simulink model "SWC_HALOUT_type"  (R2021b)
settings: Solver=FixedStepDiscrete  StartTime=0.0  StopTime=10.0  FixedStep=0.005  RelTol=1e-3
undefined symbols (not defined in the file): DIDLen_APPD, DIDLen_APPE, DIDLen_APPPedalZP, DIDLen_APSFunConfig, DIDLen_AutoLock, DIDLen_AutoWipHSpdEN, DIDLen_CALID, DIDLen_CDEODT, DIDLen_CLRDIST, DIDLen_DKCBLESta, DIDLen_DKCKey, DIDLen_DKCSta, DIDLen_DoorNFCAnchorSta, DIDLen_DRLDis, DIDLen_DynoMode, DIDLen_ECUNAME, DIDLen_FDDKCCoordXY, DIDLen_FMHTimer, DIDLen_LFLowPresThre, DIDLen_LFSensorID, DIDLen_LIDAAnchorSta, DIDLen_LRLowPresThre, DIDLen_LRSensorID, DIDLen_MILDIST, DIDLen_NUMPSATRIPSFLTMEMCLR, DIDLen_NVMPedalZP, DIDLen_OBDReq, DIDLen_ODOMETER, DIDLen_PKE, DIDLen_ProtocolId, DIDLen_PSA, DIDLen_QTYPSATRIPS, DIDLen_RFLowPresThre, DIDLen_RFSensorID, DIDLen_RRLowPresThre, DIDLen_RRSensorID, DIDLen_RUNTM, DIDLen_SensorMode, DIDLen_TestGroup, DIDLen_TireSize, DIDLen_TPMSLearnSta, DIDLen_UIDSta, DIDLen_USSConfig, DIDLen_UWBAnchorSta, DIDLen_VIN, DIDLen_VSS, DIDLen_WhlPres, DIDLen_WhlSensorBattSta, DIDLen_WhlTmp, DIDLen_WipRLSCmdCutFilter, DIDLen_WipRLSCmdHoldFilter, DIDLen_XWDMode, DIDNum_APPD, DIDNum_APPE, DIDNum_APPPedalZP, DIDNum_APSFunConfig, DIDNum_AutoLock, DIDNum_AutoWipHSpdEN, DIDNum_CALID, DIDNum_CDEODT ... (+396)
libraries: simulink x213, FVT_lib x160, hdlsllib x6, hcu_lib x5, halout x1
(part 4 of 8)

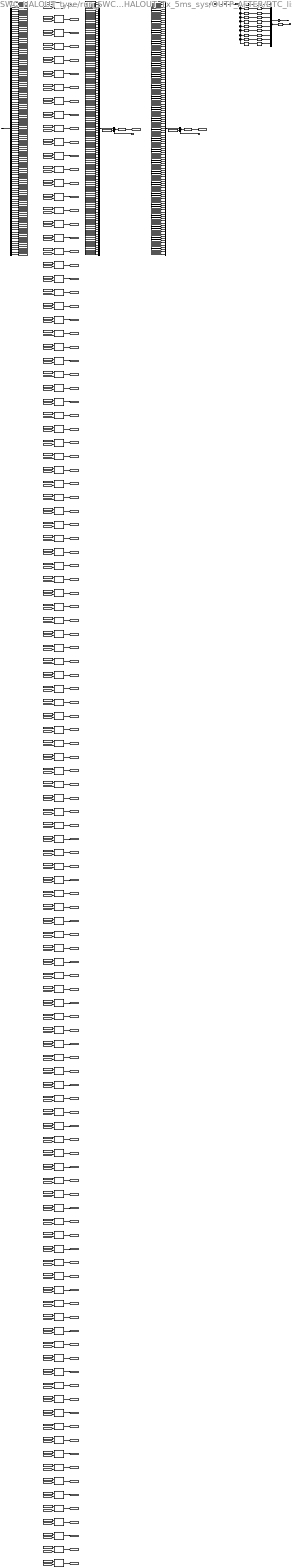
== system SWC_HALOUT_type/run_SWC_HALOUT_Tx_5ms_sys/OUTP_AFTER/DTC_list ==
  BOUTP_outputs : Inport
  BitwiseAND : simulink/Logic and Bit Operations/Bitwise Operator  logicop=AND  UseBitMask=on  BitMask=0x0001  BitMaskRealWorld=Stored Integer
  Constant : Constant  Value=DTC_D00201  OutDataTypeStr=uint16
  Constant1 : Constant  Value=DTC_D00202  OutDataTypeStr=uint16
  Constant10 : Constant  Value=DTC_10020B  OutDataTypeStr=uint16
  Constant100 : Constant  Value=DTC_900305  OutDataTypeStr=uint16
  Constant101 : Constant  Value=DTC_900253  OutDataTypeStr=uint16
  Constant102 : Constant  Value=DTC_900254  OutDataTypeStr=uint16
  Constant103 : Constant  Value=DTC_100A10  OutDataTypeStr=uint16
  Constant104 : Constant  Value=DTC_100A12  OutDataTypeStr=uint16
  Constant105 : Constant  Value=DTC_100A16  OutDataTypeStr=uint16
  Constant106 : Constant  Value=DTC_100A17  OutDataTypeStr=uint16
  Constant107 : Constant  Value=DTC_100A18  OutDataTypeStr=uint16
  Constant108 : Constant  Value=DTC_100A19  OutDataTypeStr=uint16
  Constant109 : Constant  Value=DTC_C0288F  OutDataTypeStr=uint16
  Constant11 : Constant  Value=DTC_10020C  OutDataTypeStr=uint16
  Constant110 : Constant  Value=DTC_C0378F  OutDataTypeStr=uint16
  Constant111 : Constant  Value=DTC_C0468F  OutDataTypeStr=uint16
  Constant112 : Constant  Value=DTC_C0558F  OutDataTypeStr=uint16
  Constant113 : Constant  Value=DTC_C0648F  OutDataTypeStr=uint16
  Constant114 : Constant  Value=DTC_C0808F  OutDataTypeStr=uint16
  Constant115 : Constant  Value=[0 0 0 0 0 0 0 0 0 0 0 0 0 0 0 0 0 0 0 0 0 0 0 0 0 0 0 0 0 0 0 0 0 0 0 0 0 0 0 0 0 0 0 0 0 0 0 0 0 0 0 0 0 0 0 0 0 0 0 0 0 0 0 0 0 0 0 0 0 0 0 0 0 0 0 0 0 0 0 0 0 0 0 0 0 0 0 0 0 0 0 0 0 0 0 0 0 0 0 0 0 0 0 0 0 0 0 0 0 0 0 0 0 0 0 0 0 0 0 0 0 0 0 0 0 0 0 0 0 0 0 0 0 0 0 0 0 0 0 0 0 0 0 0 0 0 0 0 0 0 0 0 0 0 0 0 0 0 0 0 0 0 0 0 0 0 0 0 0 0 0 0 0 0 0 0 0 0 0 0 0 0 0 0 0 0 0 0 0 0 0 0 0 0 0 0 0 0 0 0 0 0 0 0 0]  OutDataTypeStr=uint16
  Constant116 : DataTypeConversion
  Constant117 : Constant  Value=[0 0 0 0 0 0 0 0 0 0 0 0 0 0 0 0 0 0 0 0 0 0 0 0 0 0 0 0 0 0 0 0 0 0 0 0 0 0 0 0 0 0 0 0 0 0 0 0 0 0 0 0 0 0 0 0 0 0 0 0 0 0 0 0 0 0 0 0 0 0 0 0 0 0 0 0 0 0 0 0 0 0 0 0 0 0 0 0 0 0 0 0 0 0 0 0 0 0 0 0 0 0 0 0 0 0 0 0 0 0 0 0 0 0 0 0 0 0 0 0 0 0 0 0 0 0 0 0 0 0 0 0 0 0 0 0 0 0 0 0 0 0 0 0 0 0 0 0 0 0 0 0 0 0 0 0 0 0 0 0 0 0 0 0 0 0 0 0 0 0 0 0 0 0 0 0 0 0 0 0 0 0 0 0 0 0 0 0 0 0 0 0 0 0 0 0 0 0 0 0 0 0 0 0 0]  OutDataTypeStr=uint32
  Constant118 : DataTypeConversion
  Constant12 : Constant  Value=DTC_10020D  OutDataTypeStr=uint16
  Constant13 : Constant  Value=DTC_10020E  OutDataTypeStr=uint16
  Constant14 : Constant  Value=DTC_100210  OutDataTypeStr=uint16
  Constant15 : Constant  Value=DTC_100211  OutDataTypeStr=uint16
  Constant16 : Constant  Value=DTC_100212  OutDataTypeStr=uint16
  Constant17 : Constant  Value=DTC_100213  OutDataTypeStr=uint16
  Constant18 : Constant  Value=DTC_100214  OutDataTypeStr=uint16
  Constant19 : Constant  Value=DTC_100215  OutDataTypeStr=uint16
  Constant2 : Constant  Value=DTC_D00203  OutDataTypeStr=uint16
  Constant20 : Constant  Value=DTC_100216  OutDataTypeStr=uint16
  Constant21 : Constant  Value=DTC_100217  OutDataTypeStr=uint16
  Constant22 : Constant  Value=DTC_100218  OutDataTypeStr=uint16
  Constant23 : Constant  Value=DTC_100219  OutDataTypeStr=uint16
  Constant24 : Constant  Value=DTC_10021A  OutDataTypeStr=uint16
  Constant25 : Constant  Value=DTC_10021B  OutDataTypeStr=uint16
  Constant26 : Constant  Value=DTC_10021C  OutDataTypeStr=uint16
  Constant27 : Constant  Value=DTC_10021D  OutDataTypeStr=uint16
  Constant28 : Constant  Value=DTC_10021E  OutDataTypeStr=uint16
  Constant29 : Constant  Value=DTC_90021F  OutDataTypeStr=uint16
  Constant3 : Constant  Value=DTC_D00204  OutDataTypeStr=uint16
  Constant30 : Constant  Value=DTC_100220  OutDataTypeStr=uint16
  Constant31 : Constant  Value=DTC_100221  OutDataTypeStr=uint16
  Constant32 : Constant  Value=DTC_100223  OutDataTypeStr=uint16
  Constant33 : Constant  Value=DTC_100224  OutDataTypeStr=uint16
  Constant34 : Constant  Value=DTC_100225  OutDataTypeStr=uint16
  Constant35 : Constant  Value=DTC_100226  OutDataTypeStr=uint16
  Constant36 : Constant  Value=DTC_100227  OutDataTypeStr=uint16
  Constant37 : Constant  Value=DTC_D00228  OutDataTypeStr=uint16
  Constant38 : Constant  Value=DTC_D00229  OutDataTypeStr=uint16
  Constant39 : Constant  Value=DTC_D0022A  OutDataTypeStr=uint16
  Constant4 : Constant  Value=DTC_D00205  OutDataTypeStr=uint16
  Constant40 : Constant  Value=DTC_D0022B  OutDataTypeStr=uint16
  Constant41 : Constant  Value=DTC_D0022C  OutDataTypeStr=uint16
  Constant42 : Constant  Value=DTC_D0022D  OutDataTypeStr=uint16
  Constant43 : Constant  Value=DTC_90022F  OutDataTypeStr=uint16
  Constant44 : Constant  Value=DTC_D00230  OutDataTypeStr=uint16
  Constant45 : Constant  Value=DTC_D00231  OutDataTypeStr=uint16
  Constant46 : Constant  Value=DTC_D00232  OutDataTypeStr=uint16
  Constant47 : Constant  Value=DTC_D00234  OutDataTypeStr=uint16
  Constant48 : Constant  Value=DTC_D00235  OutDataTypeStr=uint16
  Constant49 : Constant  Value=DTC_D00236  OutDataTypeStr=uint16
  Constant5 : Constant  Value=DTC_D00206  OutDataTypeStr=uint16
  Constant50 : Constant  Value=DTC_D00237  OutDataTypeStr=uint16
  Constant51 : Constant  Value=DTC_D00238  OutDataTypeStr=uint16
  Constant52 : Constant  Value=DTC_D0023A  OutDataTypeStr=uint16
  Constant53 : Constant  Value=DTC_D0023B  OutDataTypeStr=uint16
  Constant54 : Constant  Value=DTC_D0023C  OutDataTypeStr=uint16
  Constant55 : Constant  Value=DTC_D0023D  OutDataTypeStr=uint16
  Constant56 : Constant  Value=DTC_D0023E  OutDataTypeStr=uint16
  Constant57 : Constant  Value=DTC_D00240  OutDataTypeStr=uint16
  Constant58 : Constant  Value=DTC_D00241  OutDataTypeStr=uint16
  Constant59 : Constant  Value=DTC_100242  OutDataTypeStr=uint16
  Constant6 : Constant  Value=DTC_D00207  OutDataTypeStr=uint16
  Constant60 : Constant  Value=DTC_100243  OutDataTypeStr=uint16
  Constant61 : Constant  Value=DTC_100244  OutDataTypeStr=uint16
  Constant62 : Constant  Value=DTC_100247  OutDataTypeStr=uint16
  Constant63 : Constant  Value=DTC_100248  OutDataTypeStr=uint16
  Constant64 : Constant  Value=DTC_100249  OutDataTypeStr=uint16
  Constant65 : Constant  Value=DTC_100250  OutDataTypeStr=uint16
  Constant66 : Constant  Value=DTC_100251  OutDataTypeStr=uint16
  Constant67 : Constant  Value=DTC_100252  OutDataTypeStr=uint16
  Constant68 : Constant  Value=DTC_900909  OutDataTypeStr=uint16
  Constant69 : Constant  Value=DTC_90090A  OutDataTypeStr=uint16
  Constant7 : Constant  Value=DTC_D00208  OutDataTypeStr=uint16
  Constant70 : Constant  Value=DTC_90090B  OutDataTypeStr=uint16
  Constant71 : Constant  Value=DTC_90090C  OutDataTypeStr=uint16
  Constant72 : Constant  Value=DTC_90090D  OutDataTypeStr=uint16
  Constant73 : Constant  Value=DTC_90090E  OutDataTypeStr=uint16
  Constant74 : Constant  Value=DTC_90090F  OutDataTypeStr=uint16
  Constant75 : Constant  Value=DTC_900910  OutDataTypeStr=uint16
  Constant76 : Constant  Value=DTC_900911  OutDataTypeStr=uint16
  Constant77 : Constant  Value=DTC_900912  OutDataTypeStr=uint16
  Constant78 : Constant  Value=DTC_900913  OutDataTypeStr=uint16
  Constant79 : Constant  Value=DTC_900914  OutDataTypeStr=uint16
  Constant8 : Constant  Value=DTC_D00209  OutDataTypeStr=uint16
  Constant80 : Constant  Value=DTC_500B01  OutDataTypeStr=uint16
  Constant81 : Constant  Value=DTC_500B02  OutDataTypeStr=uint16
  Constant82 : Constant  Value=DTC_500B03  OutDataTypeStr=uint16
  Constant83 : Constant  Value=DTC_500B04  OutDataTypeStr=uint16
  Constant84 : Constant  Value=DTC_500B05  OutDataTypeStr=uint16
  Constant85 : Constant  Value=DTC_500B06  OutDataTypeStr=uint16
  Constant86 : Constant  Value=DTC_500B07  OutDataTypeStr=uint16
  Constant87 : Constant  Value=DTC_500B08  OutDataTypeStr=uint16
  Constant88 : Constant  Value=DTC_500B09  OutDataTypeStr=uint16
  Constant89 : Constant  Value=DTC_500B0A  OutDataTypeStr=uint16
  Constant9 : Constant  Value=DTC_D0020A  OutDataTypeStr=uint16
  Constant90 : Constant  Value=DTC_500B0B  OutDataTypeStr=uint16
  Constant91 : Constant  Value=DTC_500B0C  OutDataTypeStr=uint16
  Constant92 : Constant  Value=DTC_500B0D  OutDataTypeStr=uint16
  Constant93 : Constant  Value=DTC_500B0E  OutDataTypeStr=uint16
  Constant94 : Constant  Value=DTC_500B0F  OutDataTypeStr=uint16
  Constant95 : Constant  Value=DTC_500B10  OutDataTypeStr=uint16
  Constant96 : Constant  Value=DTC_900301  OutDataTypeStr=uint16
  Constant97 : Constant  Value=DTC_900302  OutDataTypeStr=uint16
  Constant98 : Constant  Value=DTC_900303  OutDataTypeStr=uint16
  Constant99 : Constant  Value=DTC_900304  OutDataTypeStr=uint16
  DTCHeader{,1..9} (10 alike) : FVT_lib/hal/DTC_Header
  DTCID : Constant  Value=0xD00201
  DTCID+Status{,1..114} (115 alike) : FVT_lib/hal/DTC_ID_and_Info
  DTCID1 : Constant  Value=0xD00202
  DTCID10 : Constant  Value=0x10020B
  DTCID100 : Constant  Value=0x900305
  DTCID101 : Constant  Value=0x900253
  DTCID102 : Constant  Value=0x900254
  DTCID103 : Constant  Value=0x100A10
  DTCID104 : Constant  Value=0x100A12
  DTCID105 : Constant  Value=0x100A16
  DTCID106 : Constant  Value=0x100A17
  DTCID107 : Constant  Value=0x100A18
  DTCID108 : Constant  Value=0x100A19
  DTCID109 : Constant  Value=0xC0288F
  DTCID11 : Constant  Value=0x10020C
  DTCID110 : Constant  Value=0xC0378F
  DTCID111 : Constant  Value=0xC0468F
  DTCID112 : Constant  Value=0xC0558F
  DTCID113 : Constant  Value=0xC0648F
  DTCID114 : Constant  Value=0xC0808F
  DTCID12 : Constant  Value=0x10020D
  DTCID13 : Constant  Value=0x10020E
  DTCID14 : Constant  Value=0x100210
  DTCID15 : Constant  Value=0x100211
  DTCID16 : Constant  Value=0x100212
  DTCID17 : Constant  Value=0x100213
  DTCID18 : Constant  Value=0x100214
  DTCID19 : Constant  Value=0x100215
  DTCID2 : Constant  Value=0xD00203
  DTCID20 : Constant  Value=0x100216
  DTCID21 : Constant  Value=0x100217
  DTCID22 : Constant  Value=0x100218
  DTCID23 : Constant  Value=0x100219
  DTCID24 : Constant  Value=0x10021A
  DTCID25 : Constant  Value=0x10021B
  DTCID26 : Constant  Value=0x10021C
  DTCID27 : Constant  Value=0x10021D
  DTCID28 : Constant  Value=0x10021E
  DTCID29 : Constant  Value=0x90021F
  DTCID3 : Constant  Value=0xD00204
  DTCID30 : Constant  Value=0x100220
  DTCID31 : Constant  Value=0x100221
  DTCID32 : Constant  Value=0x100223
  DTCID33 : Constant  Value=0x100224
  DTCID34 : Constant  Value=0x100225
  DTCID35 : Constant  Value=0x100226
  DTCID36 : Constant  Value=0x100227
  DTCID37 : Constant  Value=0xD00228
  DTCID38 : Constant  Value=0xD00229
  DTCID39 : Constant  Value=0xD0022A
  DTCID4 : Constant  Value=0xD00205
  DTCID40 : Constant  Value=0xD0022B
  DTCID41 : Constant  Value=0xD0022C
  DTCID42 : Constant  Value=0xD0022D
  DTCID43 : Constant  Value=0x90022F
  DTCID44 : Constant  Value=0xD00230
  DTCID45 : Constant  Value=0xD00231
  DTCID46 : Constant  Value=0xD00232
  DTCID47 : Constant  Value=0xD00234
  DTCID48 : Constant  Value=0xD00235
  DTCID49 : Constant  Value=0xD00236
  DTCID5 : Constant  Value=0xD00206
  DTCID50 : Constant  Value=0xD00237
  DTCID51 : Constant  Value=0xD00238
  DTCID52 : Constant  Value=0xD0023A
  DTCID53 : Constant  Value=0xD0023B
  DTCID54 : Constant  Value=0xD0023C
  DTCID55 : Constant  Value=0xD0023D
  DTCID56 : Constant  Value=0xD0023E
  DTCID57 : Constant  Value=0xD00240
  DTCID58 : Constant  Value=0xD00241
  DTCID59 : Constant  Value=0x100242
  DTCID6 : Constant  Value=0xD00207
  DTCID60 : Constant  Value=0x100243
  DTCID61 : Constant  Value=0x100244
  DTCID62 : Constant  Value=0x100247
  DTCID63 : Constant  Value=0x100248
  DTCID64 : Constant  Value=0x100249
  DTCID65 : Constant  Value=0x100250
  DTCID66 : Constant  Value=0x100251
  DTCID67 : Constant  Value=0x100252
  DTCID68 : Constant  Value=0x900909
  DTCID69 : Constant  Value=0x90090A
  DTCID7 : Constant  Value=0xD00208
  DTCID70 : Constant  Value=0x90090B
  DTCID71 : Constant  Value=0x90090C
  DTCID72 : Constant  Value=0x90090D
  DTCID73 : Constant  Value=0x90090E
  DTCID74 : Constant  Value=0x90090F
  DTCID75 : Constant  Value=0x900910
  DTCID76 : Constant  Value=0x900911
  DTCID77 : Constant  Value=0x900912
  DTCID78 : Constant  Value=0x900913
  DTCID79 : Constant  Value=0x900914
  DTCID8 : Constant  Value=0xD00209
  DTCID80 : Constant  Value=0x500B01
  DTCID81 : Constant  Value=0x500B02
  DTCID82 : Constant  Value=0x500B03
  DTCID83 : Constant  Value=0x500B04
  DTCID84 : Constant  Value=0x500B05
  DTCID85 : Constant  Value=0x500B06
  DTCID86 : Constant  Value=0x500B07
  DTCID87 : Constant  Value=0x500B08
  DTCID88 : Constant  Value=0x500B09
  DTCID89 : Constant  Value=0x500B0A
  DTCID9 : Constant  Value=0xD0020A
  DTCID90 : Constant  Value=0x500B0B
  DTCID91 : Constant  Value=0x500B0C
  DTCID92 : Constant  Value=0x500B0D
  DTCID93 : Constant  Value=0x500B0E
  DTCID94 : Constant  Value=0x500B0F
  DTCID95 : Constant  Value=0x500B10
  DTCID96 : Constant  Value=0x900301
  DTCID97 : Constant  Value=0x900302
  DTCID98 : Constant  Value=0x900303
  DTCID99 : Constant  Value=0x900304
  Mux : Mux  Inputs=115
  Mux1 : Mux  Inputs=2
  Mux2 : Mux  Inputs=115
  Mux3 : Mux  Inputs=2
  Mux4 : Mux  Inputs=10
  OR : Logic  Operator=OR  Inputs=1  AllPortsSameDT=off  OutDataTypeStr=boolean
  Selector : Selector  InputPortWidth=320  IndexOptions=Index vector (dialog)  Indices=[1:32]  OutputSizes=1
  Selector1 : Selector  InputPortWidth=320  IndexOptions=Index vector (dialog)  Indices=[33:64]  OutputSizes=1
  Selector2 : Selector  InputPortWidth=320  IndexOptions=Index vector (dialog)  Indices=[65:96]  OutputSizes=1
  Selector3 : Selector  InputPortWidth=320  IndexOptions=Index vector (dialog)  Indices=[97:128]  OutputSizes=1
  Selector4 : Selector  InputPortWidth=320  IndexOptions=Index vector (dialog)  Indices=[129:160]  OutputSizes=1
  Selector5 : Selector  InputPortWidth=320  IndexOptions=Index vector (dialog)  Indices=[161:192]  OutputSizes=1
  Selector6 : Selector  InputPortWidth=320  IndexOptions=Index vector (dialog)  Indices=[193:224]  OutputSizes=1
  Selector7 : Selector  InputPortWidth=320  IndexOptions=Index vector (dialog)  Indices=[225:256]  OutputSizes=1
  Selector8 : Selector  InputPortWidth=320  IndexOptions=Index vector (dialog)  Indices=[257:288]  OutputSizes=1
  Selector9 : Selector  InputPortWidth=320  IndexOptions=Index vector (dialog)  Indices=[289:320]  OutputSizes=1
  UnitConverter : DataTypeConversion
  bus_selector : BusSelector  OutputSignals=VOUTP_5vAPS1PwrErrDTC_raw32,VOUTP_5vAPS2PwrErrDTC_raw32,VOUTP_ACCAccelCmdErrDetDTC_raw32,VOUTP_APS1SigOoRDTC_raw32,VOUTP_APS2SigOoRDTC_raw32,VOUTP_APSCorrErrDTC_raw32,VOUTP_BMSRdyDTC_raw32,VOUTP_BMSSigErrDetDTC_raw32,VOUTP_BrkSWErrDTC_raw32,VOUTP_BrkSWNoBacDTC_raw32,VOUTP_C1ABM1CSDTC_raw32,VOUTP_C1ABM1LCDTC_raw32,VOUTP_C1ABM1RCDTC_raw32,VOUTP_C3BMS1CSDTC_raw32,VOUTP_C3BMS1LCDTC_raw32,VOUTP_C3BMS1RCDTC_raw32,VOUTP_C3BMS6CSDTC_raw32,VOUTP_C3BMS6LCDTC_raw32,VOUTP_C3BMS6RCDTC_raw32,VOUTP_C3CCU1CSDTC_raw32,VOUTP_C3CCU1LCDTC_raw32,VOUTP_C3CCU1RCDTC_raw32,VOUTP_C3CCU2CSDTC_raw32,VOUTP_C3CCU2LCDTC_raw32,VOUTP_C3CCU2RCDTC_raw32,VOUTP_CAN1BusErrorDTC_raw32,VOUTP_CAN2BusErrorDTC_raw32,VOUTP_CAN3BusErrorDTC_raw32,VOUTP_CAN4BusErrorDTC_raw32,VOUTP_CAN5BusErrorDTC_raw32,VOUTP_CAN6BusErrorDTC_raw32,VOUTP_CCUSigErrDetDTC_raw32,VOUTP_DCDC4PreDTC_raw32,VOUTP_DCDCDisDTC_raw32,VOUTP_DCDCEnaDTC_raw32,VOUTP_DiagFLTSDTC_raw32,VOUTP_DiagFRTSDTC_raw32,VOUTP_DiagHCrashDTC_raw32,VOUTP_DiagRLTSDTC_raw32,VOUTP_DiagRRTSDTC_raw32,VOUTP_DrStSWDTC_raw32,VOUTP_EPBLockTODTC_raw32,VOUTP_EPBUnlockTODTC_raw32,VOUTP_ESC1CSErrDTC_raw32,VOUTP_ESC1NoComDTC_raw32,VOUTP_ESC1RCErrDTC_raw32,VOUTP_ESC5CSErrDTC_raw32,VOUTP_ESC5NoComDTC_raw32,VOUTP_ESC5RCErrDTC_raw32,VOUTP_FCLUSSDTC_raw32,VOUTP_FCMACCSigErrDetDTC_raw32,VOUTP_FCRUSSDTC_raw32,VOUTP_FLDoorSWDTC_raw32,VOUTP_FLLUSSDTC_raw32,VOUTP_FLRUSSDTC_raw32,VOUTP_FMLUSSDTC_raw32,VOUTP_FMRUSSDTC_raw32,VOUTP_FRDoorSWDTC_raw32,VOUTP_FrMCUSigErrDetDTC_raw32,VOUTP_FrMCUTqErrDTC_raw32,VOUTP_HVB4PreDTC_raw32,VOUTP_HVRlyCloDTC_raw32,VOUTP_HVRlyOpDTC_raw32,VOUTP_HiLvSaChkDTC_raw32,VOUTP_HoodSWDTC_raw32,VOUTP_IniLVLoDTC_raw32,VOUTP_KeyAuthDTC_raw32,VOUTP_LFBatwarnDTC_raw32,VOUTP_LFPressIndiDTC_raw32,VOUTP_LFSensorFailDTC_raw32,VOUTP_LFWheelTmpHighDTC_raw32,VOUTP_LRBatwarnDTC_raw32,VOUTP_LRPressIndiDTC_raw32,VOUTP_LRSensorFailDTC_raw32,VOUTP_LRWheelTmpHighDTC_raw32,VOUTP_LVSupHiDTC_raw32,VOUTP_LVSupLoDTC_raw32,VOUTP_Lv1ErrDTC_raw32,VOUTP_Lv2ErrDTC_raw32,VOUTP_Lv3ErrDTC_raw32,VOUTP_Lv4ErrDTC_raw32,VOUTP_MCU4PreDTC_raw32,VOUTP_MCUActDTC_raw32,VOUTP_MCUDisDTC_raw32,VOUTP_MCUF1CSErrDTC_raw32,VOUTP_MCUF1NoComDTC_raw32,VOUTP_MCUF1RCErrDTC_raw32,VOUTP_MCUR1CSErrDTC_raw32,VOUTP_MCUR1NoComDTC_raw32,VOUTP_MCUR1RCErrDTC_raw32,VOUTP_MidLvSaChkDTC_raw32,VOUTP_OBC4PreDTC_raw32,VOUTP_ONtoRdyDTC_raw32,VOUTP_RCLUSSDTC_raw32,VOUTP_RCRUSSDTC_raw32,VOUTP_RFBatwarnDTC_raw32,VOUTP_RFPressIndiDTC_raw32,VOUTP_RFSensorFailDTC_raw32,VOUTP_RFWheelTmpHighDTC_raw32,VOUTP_RLDoorSWDTC_raw32,VOUTP_RLLUSSDTC_raw32,VOUTP_RLRUSSDTC_raw32,VOUTP_RMLUSSDTC_raw32,VOUTP_RMRUSSDTC_raw32,VOUTP_RRBatwarnDTC_raw32,VOUTP_RRDoorSWDTC_raw32,VOUTP_RRPressIndiDTC_raw32,VOUTP_RRSensorFailDTC_raw32,VOUTP_RRWheelTmpHighDTC_raw32,VOUTP_RrMCUSigErrDetDTC_raw32,VOUTP_RrMCUTqErrDTC_raw32,VOUTP_Shifter1CSErrDTC_raw32,VOUTP_Shifter1NoComDTC_raw32,VOUTP_Shifter1RCErrDTC_raw32,VOUTP_TailgaSWDTC_raw32
  detect_change : simulink/Logic and Bit Operations/Detect Change  vinit=0  OutDataTypeStr=boolean
  Trigger : Outport
  Header_Array : Outport  Port=2
  DTC_Constant_Array : Outport  Port=3
  DTC_Array : Outport  Port=4
  wires:
  BOUTP_outputs/1 -> bus_selector/1
  bus_selector/1 -> [VOUTP_5vAPS1PwrErrDTC_raw32]  "<VOUTP_5vAPS1PwrErrDTC_raw32>"
  bus_selector/2 -> [VOUTP_5vAPS2PwrErrDTC_raw32]  "<VOUTP_5vAPS2PwrErrDTC_raw32>"
  bus_selector/3 -> [VOUTP_ACCAccelCmdErrDetDTC_raw32]  "<VOUTP_ACCAccelCmdErrDetDTC_raw32>"
  bus_selector/4 -> [VOUTP_APS1SigOoRDTC_raw32]  "<VOUTP_APS1SigOoRDTC_raw32>"
  bus_selector/5 -> [VOUTP_APS2SigOoRDTC_raw32]  "<VOUTP_APS2SigOoRDTC_raw32>"
  bus_selector/6 -> [VOUTP_APSCorrErrDTC_raw32]  "<VOUTP_APSCorrErrDTC_raw32>"
  bus_selector/7 -> [VOUTP_BMSRdyDTC_raw32]  "<VOUTP_BMSRdyDTC_raw32>"
  bus_selector/8 -> [VOUTP_BMSSigErrDetDTC_raw32]  "<VOUTP_BMSSigErrDetDTC_raw32>"
  bus_selector/9 -> [VOUTP_BrkSWErrDTC_raw32]  "<VOUTP_BrkSWErrDTC_raw32>"
  bus_selector/10 -> [VOUTP_BrkSWNoBacDTC_raw32]  "<VOUTP_BrkSWNoBacDTC_raw32>"
  bus_selector/11 -> [VOUTP_C1ABM1CSDTC_raw32]  "<VOUTP_C1ABM1CSDTC_raw32>"
  bus_selector/12 -> [VOUTP_C1ABM1LCDTC_raw32]  "<VOUTP_C1ABM1LCDTC_raw32>"
  bus_selector/13 -> [VOUTP_C1ABM1RCDTC_raw32]  "<VOUTP_C1ABM1RCDTC_raw32>"
  bus_selector/14 -> [VOUTP_C3BMS1CSDTC_raw32]  "<VOUTP_C3BMS1CSDTC_raw32>"
  bus_selector/15 -> [VOUTP_C3BMS1LCDTC_raw32]  "<VOUTP_C3BMS1LCDTC_raw32>"
  bus_selector/16 -> [VOUTP_C3BMS1RCDTC_raw32]  "<VOUTP_C3BMS1RCDTC_raw32>"
  bus_selector/17 -> [VOUTP_C3BMS6CSDTC_raw32]  "<VOUTP_C3BMS6CSDTC_raw32>"
  bus_selector/18 -> [VOUTP_C3BMS6LCDTC_raw32]  "<VOUTP_C3BMS6LCDTC_raw32>"
  bus_selector/19 -> [VOUTP_C3BMS6RCDTC_raw32]  "<VOUTP_C3BMS6RCDTC_raw32>"
  bus_selector/20 -> [VOUTP_C3CCU1CSDTC_raw32]  "<VOUTP_C3CCU1CSDTC_raw32>"
  bus_selector/21 -> [VOUTP_C3CCU1LCDTC_raw32]  "<VOUTP_C3CCU1LCDTC_raw32>"
  bus_selector/22 -> [VOUTP_C3CCU1RCDTC_raw32]  "<VOUTP_C3CCU1RCDTC_raw32>"
  bus_selector/23 -> [VOUTP_C3CCU2CSDTC_raw32]  "<VOUTP_C3CCU2CSDTC_raw32>"
  bus_selector/24 -> [VOUTP_C3CCU2LCDTC_raw32]  "<VOUTP_C3CCU2LCDTC_raw32>"
  bus_selector/25 -> [VOUTP_C3CCU2RCDTC_raw32]  "<VOUTP_C3CCU2RCDTC_raw32>"
  bus_selector/26 -> [VOUTP_CAN1BusErrorDTC_raw32]  "<VOUTP_CAN1BusErrorDTC_raw32>"
  bus_selector/27 -> [VOUTP_CAN2BusErrorDTC_raw32]  "<VOUTP_CAN2BusErrorDTC_raw32>"
  bus_selector/28 -> [VOUTP_CAN3BusErrorDTC_raw32]  "<VOUTP_CAN3BusErrorDTC_raw32>"
  bus_selector/29 -> [VOUTP_CAN4BusErrorDTC_raw32]  "<VOUTP_CAN4BusErrorDTC_raw32>"
  bus_selector/30 -> [VOUTP_CAN5BusErrorDTC_raw32]  "<VOUTP_CAN5BusErrorDTC_raw32>"
  bus_selector/31 -> [VOUTP_CAN6BusErrorDTC_raw32]  "<VOUTP_CAN6BusErrorDTC_raw32>"
  bus_selector/32 -> [VOUTP_CCUSigErrDetDTC_raw32]  "<VOUTP_CCUSigErrDetDTC_raw32>"
  bus_selector/33 -> [VOUTP_DCDC4PreDTC_raw32]  "<VOUTP_DCDC4PreDTC_raw32>"
  bus_selector/34 -> [VOUTP_DCDCDisDTC_raw32]  "<VOUTP_DCDCDisDTC_raw32>"
  bus_selector/35 -> [VOUTP_DCDCEnaDTC_raw32]  "<VOUTP_DCDCEnaDTC_raw32>"
  bus_selector/36 -> [VOUTP_DiagFLTSDTC_raw32]  "<VOUTP_DiagFLTSDTC_raw32>"
  bus_selector/37 -> [VOUTP_DiagFRTSDTC_raw32]  "<VOUTP_DiagFRTSDTC_raw32>"
  bus_selector/38 -> [VOUTP_DiagHCrashDTC_raw32]  "<VOUTP_DiagHCrashDTC_raw32>"
  bus_selector/39 -> [VOUTP_DiagRLTSDTC_raw32]  "<VOUTP_DiagRLTSDTC_raw32>"
  bus_selector/40 -> [VOUTP_DiagRRTSDTC_raw32]  "<VOUTP_DiagRRTSDTC_raw32>"
  bus_selector/41 -> [VOUTP_DrStSWDTC_raw32]  "<VOUTP_DrStSWDTC_raw32>"
  bus_selector/42 -> [VOUTP_EPBLockTODTC_raw32]  "<VOUTP_EPBLockTODTC_raw32>"
  bus_selector/43 -> [VOUTP_EPBUnlockTODTC_raw32]  "<VOUTP_EPBUnlockTODTC_raw32>"
  bus_selector/44 -> [VOUTP_ESC1CSErrDTC_raw32]  "<VOUTP_ESC1CSErrDTC_raw32>"
  bus_selector/45 -> [VOUTP_ESC1NoComDTC_raw32]  "<VOUTP_ESC1NoComDTC_raw32>"
  bus_selector/46 -> [VOUTP_ESC1RCErrDTC_raw32]  "<VOUTP_ESC1RCErrDTC_raw32>"
  bus_selector/47 -> [VOUTP_ESC5CSErrDTC_raw32]  "<VOUTP_ESC5CSErrDTC_raw32>"
  bus_selector/48 -> [VOUTP_ESC5NoComDTC_raw32]  "<VOUTP_ESC5NoComDTC_raw32>"
  bus_selector/49 -> [VOUTP_ESC5RCErrDTC_raw32]  "<VOUTP_ESC5RCErrDTC_raw32>"
  bus_selector/50 -> [VOUTP_FCLUSSDTC_raw32]  "<VOUTP_FCLUSSDTC_raw32>"
  bus_selector/51 -> [VOUTP_FCMACCSigErrDetDTC_raw32]  "<VOUTP_FCMACCSigErrDetDTC_raw32>"
  bus_selector/52 -> [VOUTP_FCRUSSDTC_raw32]  "<VOUTP_FCRUSSDTC_raw32>"
  bus_selector/53 -> [VOUTP_FLDoorSWDTC_raw32]  "<VOUTP_FLDoorSWDTC_raw32>"
  bus_selector/54 -> [VOUTP_FLLUSSDTC_raw32]  "<VOUTP_FLLUSSDTC_raw32>"
  bus_selector/55 -> [VOUTP_FLRUSSDTC_raw32]  "<VOUTP_FLRUSSDTC_raw32>"
  bus_selector/56 -> [VOUTP_FMLUSSDTC_raw32]  "<VOUTP_FMLUSSDTC_raw32>"
  bus_selector/57 -> [VOUTP_FMRUSSDTC_raw32]  "<VOUTP_FMRUSSDTC_raw32>"
  bus_selector/58 -> [VOUTP_FRDoorSWDTC_raw32]  "<VOUTP_FRDoorSWDTC_raw32>"
  bus_selector/59 -> [VOUTP_FrMCUSigErrDetDTC_raw32]  "<VOUTP_FrMCUSigErrDetDTC_raw32>"
  bus_selector/60 -> [VOUTP_FrMCUTqErrDTC_raw32]  "<VOUTP_FrMCUTqErrDTC_raw32>"
  bus_selector/61 -> [VOUTP_HVB4PreDTC_raw32]  "<VOUTP_HVB4PreDTC_raw32>"
  bus_selector/62 -> [VOUTP_HVRlyCloDTC_raw32]  "<VOUTP_HVRlyCloDTC_raw32>"
  bus_selector/63 -> [VOUTP_HVRlyOpDTC_raw32]  "<VOUTP_HVRlyOpDTC_raw32>"
  bus_selector/64 -> [VOUTP_HiLvSaChkDTC_raw32]  "<VOUTP_HiLvSaChkDTC_raw32>"
  bus_selector/65 -> [VOUTP_HoodSWDTC_raw32]  "<VOUTP_HoodSWDTC_raw32>"
  bus_selector/66 -> [VOUTP_IniLVLoDTC_raw32]  "<VOUTP_IniLVLoDTC_raw32>"
  bus_selector/67 -> [VOUTP_KeyAuthDTC_raw32]  "<VOUTP_KeyAuthDTC_raw32>"
  bus_selector/68 -> [VOUTP_LFBatwarnDTC_raw32]  "<VOUTP_LFBatwarnDTC_raw32>"
  bus_selector/69 -> [VOUTP_LFPressIndiDTC_raw32]  "<VOUTP_LFPressIndiDTC_raw32>"
  bus_selector/70 -> [VOUTP_LFSensorFailDTC_raw32]  "<VOUTP_LFSensorFailDTC_raw32>"
  bus_selector/71 -> [VOUTP_LFWheelTmpHighDTC_raw32]  "<VOUTP_LFWheelTmpHighDTC_raw32>"
  bus_selector/72 -> [VOUTP_LRBatwarnDTC_raw32]  "<VOUTP_LRBatwarnDTC_raw32>"
  bus_selector/73 -> [VOUTP_LRPressIndiDTC_raw32]  "<VOUTP_LRPressIndiDTC_raw32>"
  bus_selector/74 -> [VOUTP_LRSensorFailDTC_raw32]  "<VOUTP_LRSensorFailDTC_raw32>"
  bus_selector/75 -> [VOUTP_LRWheelTmpHighDTC_raw32]  "<VOUTP_LRWheelTmpHighDTC_raw32>"
  bus_selector/76 -> [VOUTP_LVSupHiDTC_raw32]  "<VOUTP_LVSupHiDTC_raw32>"
  bus_selector/77 -> [VOUTP_LVSupLoDTC_raw32]  "<VOUTP_LVSupLoDTC_raw32>"
  bus_selector/78 -> [VOUTP_Lv1ErrDTC_raw32]  "<VOUTP_Lv1ErrDTC_raw32>"
  bus_selector/79 -> [VOUTP_Lv2ErrDTC_raw32]  "<VOUTP_Lv2ErrDTC_raw32>"
  bus_selector/80 -> [VOUTP_Lv3ErrDTC_raw32]  "<VOUTP_Lv3ErrDTC_raw32>"
  bus_selector/81 -> [VOUTP_Lv4ErrDTC_raw32]  "<VOUTP_Lv4ErrDTC_raw32>"
  bus_selector/82 -> [VOUTP_MCU4PreDTC_raw32]  "<VOUTP_MCU4PreDTC_raw32>"
  bus_selector/83 -> [VOUTP_MCUActDTC_raw32]  "<VOUTP_MCUActDTC_raw32>"
  bus_selector/84 -> [VOUTP_MCUDisDTC_raw32]  "<VOUTP_MCUDisDTC_raw32>"
  bus_selector/85 -> [VOUTP_MCUF1CSErrDTC_raw32]  "<VOUTP_MCUF1CSErrDTC_raw32>"
  bus_selector/86 -> [VOUTP_MCUF1NoComDTC_raw32]  "<VOUTP_MCUF1NoComDTC_raw32>"
  bus_selector/87 -> [VOUTP_MCUF1RCErrDTC_raw32]  "<VOUTP_MCUF1RCErrDTC_raw32>"
  bus_selector/88 -> [VOUTP_MCUR1CSErrDTC_raw32]  "<VOUTP_MCUR1CSErrDTC_raw32>"
  bus_selector/89 -> [VOUTP_MCUR1NoComDTC_raw32]  "<VOUTP_MCUR1NoComDTC_raw32>"
  bus_selector/90 -> [VOUTP_MCUR1RCErrDTC_raw32]  "<VOUTP_MCUR1RCErrDTC_raw32>"
  bus_selector/91 -> [VOUTP_MidLvSaChkDTC_raw32]  "<VOUTP_MidLvSaChkDTC_raw32>"
  bus_selector/92 -> [VOUTP_OBC4PreDTC_raw32]  "<VOUTP_OBC4PreDTC_raw32>"
  bus_selector/93 -> [VOUTP_ONtoRdyDTC_raw32]  "<VOUTP_ONtoRdyDTC_raw32>"
  bus_selector/94 -> [VOUTP_RCLUSSDTC_raw32]  "<VOUTP_RCLUSSDTC_raw32>"
  bus_selector/95 -> [VOUTP_RCRUSSDTC_raw32]  "<VOUTP_RCRUSSDTC_raw32>"
  bus_selector/96 -> [VOUTP_RFBatwarnDTC_raw32]  "<VOUTP_RFBatwarnDTC_raw32>"
  bus_selector/97 -> [VOUTP_RFPressIndiDTC_raw32]  "<VOUTP_RFPressIndiDTC_raw32>"
  bus_selector/98 -> [VOUTP_RFSensorFailDTC_raw32]  "<VOUTP_RFSensorFailDTC_raw32>"
  bus_selector/99 -> [VOUTP_RFWheelTmpHighDTC_raw32]  "<VOUTP_RFWheelTmpHighDTC_raw32>"
  bus_selector/100 -> [VOUTP_RLDoorSWDTC_raw32]  "<VOUTP_RLDoorSWDTC_raw32>"
  bus_selector/101 -> [VOUTP_RLLUSSDTC_raw32]  "<VOUTP_RLLUSSDTC_raw32>"
  bus_selector/102 -> [VOUTP_RLRUSSDTC_raw32]  "<VOUTP_RLRUSSDTC_raw32>"
  bus_selector/103 -> [VOUTP_RMLUSSDTC_raw32]  "<VOUTP_RMLUSSDTC_raw32>"
  bus_selector/104 -> [VOUTP_RMRUSSDTC_raw32]  "<VOUTP_RMRUSSDTC_raw32>"
  bus_selector/105 -> [VOUTP_RRBatwarnDTC_raw32]  "<VOUTP_RRBatwarnDTC_raw32>"
  bus_selector/106 -> [VOUTP_RRDoorSWDTC_raw32]  "<VOUTP_RRDoorSWDTC_raw32>"
  bus_selector/107 -> [VOUTP_RRPressIndiDTC_raw32]  "<VOUTP_RRPressIndiDTC_raw32>"
  bus_selector/108 -> [VOUTP_RRSensorFailDTC_raw32]  "<VOUTP_RRSensorFailDTC_raw32>"
  bus_selector/109 -> [VOUTP_RRWheelTmpHighDTC_raw32]  "<VOUTP_RRWheelTmpHighDTC_raw32>"
  bus_selector/110 -> [VOUTP_RrMCUSigErrDetDTC_raw32]  "<VOUTP_RrMCUSigErrDetDTC_raw32>"
  bus_selector/111 -> [VOUTP_RrMCUTqErrDTC_raw32]  "<VOUTP_RrMCUTqErrDTC_raw32>"
  bus_selector/112 -> [VOUTP_Shifter1CSErrDTC_raw32]  "<VOUTP_Shifter1CSErrDTC_raw32>"
  bus_selector/113 -> [VOUTP_Shifter1NoComDTC_raw32]  "<VOUTP_Shifter1NoComDTC_raw32>"
  bus_selector/114 -> [VOUTP_Shifter1RCErrDTC_raw32]  "<VOUTP_Shifter1RCErrDTC_raw32>"
  bus_selector/115 -> [VOUTP_TailgaSWDTC_raw32]  "<VOUTP_TailgaSWDTC_raw32>"
  DTCID/1 -> DTCID+Status/1
  [VOUTP_C3BMS6RCDTC_raw32] -> DTCID+Status/2
  DTCID+Status/1 -> [DTC_raw0]
  DTCID1/1 -> DTCID+Status1/1
  [VOUTP_C3BMS6CSDTC_raw32] -> DTCID+Status1/2
  DTCID+Status1/1 -> [DTC_raw1]
  DTCID2/1 -> DTCID+Status2/1
  [VOUTP_C3BMS1RCDTC_raw32] -> DTCID+Status2/2
  DTCID+Status2/1 -> [DTC_raw2]
  DTCID3/1 -> DTCID+Status3/1
  [VOUTP_C3BMS1CSDTC_raw32] -> DTCID+Status3/2
  DTCID+Status3/1 -> [DTC_raw3]
  DTCID4/1 -> DTCID+Status4/1
  [VOUTP_C3CCU1RCDTC_raw32] -> DTCID+Status4/2
  DTCID+Status4/1 -> [DTC_raw4]
  DTCID5/1 -> DTCID+Status5/1
  [VOUTP_C3CCU1CSDTC_raw32] -> DTCID+Status5/2
  DTCID+Status5/1 -> [DTC_raw5]
  DTCID6/1 -> DTCID+Status6/1
  [VOUTP_C3CCU2RCDTC_raw32] -> DTCID+Status6/2
  DTCID+Status6/1 -> [DTC_raw6]
  DTCID7/1 -> DTCID+Status7/1
  [VOUTP_C3CCU2CSDTC_raw32] -> DTCID+Status7/2
  DTCID+Status7/1 -> [DTC_raw7]
  DTCID8/1 -> DTCID+Status8/1
  [VOUTP_C1ABM1RCDTC_raw32] -> DTCID+Status8/2
  DTCID+Status8/1 -> [DTC_raw8]
  DTCID9/1 -> DTCID+Status9/1
  [VOUTP_C1ABM1CSDTC_raw32] -> DTCID+Status9/2
  DTCID+Status9/1 -> [DTC_raw9]
  DTCID10/1 -> DTCID+Status10/1
  [VOUTP_Lv1ErrDTC_raw32] -> DTCID+Status10/2
  DTCID+Status10/1 -> [DTC_raw10]
  DTCID11/1 -> DTCID+Status11/1
  [VOUTP_Lv2ErrDTC_raw32] -> DTCID+Status11/2
  DTCID+Status11/1 -> [DTC_raw11]
  DTCID12/1 -> DTCID+Status12/1
  [VOUTP_Lv3ErrDTC_raw32] -> DTCID+Status12/2
  DTCID+Status12/1 -> [DTC_raw12]
  DTCID13/1 -> DTCID+Status13/1
  [VOUTP_Lv4ErrDTC_raw32] -> DTCID+Status13/2
  DTCID+Status13/1 -> [DTC_raw13]
  DTCID14/1 -> DTCID+Status14/1
  [VOUTP_IniLVLoDTC_raw32] -> DTCID+Status14/2
  DTCID+Status14/1 -> [DTC_raw14]
  DTCID15/1 -> DTCID+Status15/1
  [VOUTP_LVSupHiDTC_raw32] -> DTCID+Status15/2
  DTCID+Status15/1 -> [DTC_raw15]
  DTCID16/1 -> DTCID+Status16/1
  [VOUTP_LVSupLoDTC_raw32] -> DTCID+Status16/2
  DTCID+Status16/1 -> [DTC_raw16]
  DTCID17/1 -> DTCID+Status17/1
  [VOUTP_HVB4PreDTC_raw32] -> DTCID+Status17/2
  DTCID+Status17/1 -> [DTC_raw17]
  DTCID18/1 -> DTCID+Status18/1
  [VOUTP_MCU4PreDTC_raw32] -> DTCID+Status18/2
  DTCID+Status18/1 -> [DTC_raw18]
  DTCID19/1 -> DTCID+Status19/1
  [VOUTP_DCDC4PreDTC_raw32] -> DTCID+Status19/2
  DTCID+Status19/1 -> [DTC_raw19]
  DTCID20/1 -> DTCID+Status20/1
  [VOUTP_HVRlyCloDTC_raw32] -> DTCID+Status20/2
  DTCID+Status20/1 -> [DTC_raw20]
  DTCID21/1 -> DTCID+Status21/1
  [VOUTP_BMSRdyDTC_raw32] -> DTCID+Status21/2
  DTCID+Status21/1 -> [DTC_raw21]
  DTCID22/1 -> DTCID+Status22/1
  [VOUTP_DCDCEnaDTC_raw32] -> DTCID+Status22/2
  DTCID+Status22/1 -> [DTC_raw22]
  DTCID23/1 -> DTCID+Status23/1
  [VOUTP_HiLvSaChkDTC_raw32] -> DTCID+Status23/2
  DTCID+Status23/1 -> [DTC_raw23]
  DTCID24/1 -> DTCID+Status24/1
  [VOUTP_MidLvSaChkDTC_raw32] -> DTCID+Status24/2
  DTCID+Status24/1 -> [DTC_raw24]
  DTCID25/1 -> DTCID+Status25/1
  [VOUTP_MCUDisDTC_raw32] -> DTCID+Status25/2
  DTCID+Status25/1 -> [DTC_raw25]
  DTCID26/1 -> DTCID+Status26/1
  [VOUTP_DCDCDisDTC_raw32] -> DTCID+Status26/2
  DTCID+Status26/1 -> [DTC_raw26]
  DTCID27/1 -> DTCID+Status27/1
  [VOUTP_HVRlyOpDTC_raw32] -> DTCID+Status27/2
  DTCID+Status27/1 -> [DTC_raw27]
  DTCID28/1 -> DTCID+Status28/1
  [VOUTP_MCUActDTC_raw32] -> DTCID+Status28/2
  DTCID+Status28/1 -> [DTC_raw28]
  DTCID29/1 -> DTCID+Status29/1
  [VOUTP_OBC4PreDTC_raw32] -> DTCID+Status29/2
  DTCID+Status29/1 -> [DTC_raw29]
  DTCID30/1 -> DTCID+Status30/1
  [VOUTP_BrkSWErrDTC_raw32] -> DTCID+Status30/2
  DTCID+Status30/1 -> [DTC_raw30]
  DTCID31/1 -> DTCID+Status31/1
  [VOUTP_BrkSWNoBacDTC_raw32] -> DTCID+Status31/2
  DTCID+Status31/1 -> [DTC_raw31]
  DTCID32/1 -> DTCID+Status32/1
  [VOUTP_DrStSWDTC_raw32] -> DTCID+Status32/2
  DTCID+Status32/1 -> [DTC_raw32]
  DTCID33/1 -> DTCID+Status33/1
  [VOUTP_FLDoorSWDTC_raw32] -> DTCID+Status33/2
  DTCID+Status33/1 -> [DTC_raw33]
  DTCID34/1 -> DTCID+Status34/1
  [VOUTP_FRDoorSWDTC_raw32] -> DTCID+Status34/2
  DTCID+Status34/1 -> [DTC_raw34]
  DTCID35/1 -> DTCID+Status35/1
  [VOUTP_RLDoorSWDTC_raw32] -> DTCID+Status35/2
  DTCID+Status35/1 -> [DTC_raw35]
  DTCID36/1 -> DTCID+Status36/1
  [VOUTP_RRDoorSWDTC_raw32] -> DTCID+Status36/2
  DTCID+Status36/1 -> [DTC_raw36]
  DTCID37/1 -> DTCID+Status37/1
  [VOUTP_C3BMS6LCDTC_raw32] -> DTCID+Status37/2
  DTCID+Status37/1 -> [DTC_raw37]
  DTCID38/1 -> DTCID+Status38/1
  [VOUTP_C3BMS1LCDTC_raw32] -> DTCID+Status38/2
  DTCID+Status38/1 -> [DTC_raw38]
  DTCID39/1 -> DTCID+Status39/1
  [VOUTP_C3CCU1LCDTC_raw32] -> DTCID+Status39/2
  DTCID+Status39/1 -> [DTC_raw39]
  DTCID40/1 -> DTCID+Status40/1
  [VOUTP_C3CCU2LCDTC_raw32] -> DTCID+Status40/2
  DTCID+Status40/1 -> [DTC_raw40]
  DTCID41/1 -> DTCID+Status41/1
  [VOUTP_C1ABM1LCDTC_raw32] -> DTCID+Status41/2
  DTCID+Status41/1 -> [DTC_raw41]
  DTCID42/1 -> DTCID+Status42/1
  [VOUTP_KeyAuthDTC_raw32] -> DTCID+Status42/2
  DTCID+Status42/1 -> [DTC_raw42]
  DTCID43/1 -> DTCID+Status43/1
  [VOUTP_ONtoRdyDTC_raw32] -> DTCID+Status43/2
  DTCID+Status43/1 -> [DTC_raw43]
  DTCID44/1 -> DTCID+Status44/1
  [VOUTP_MCUR1NoComDTC_raw32] -> DTCID+Status44/2
  DTCID+Status44/1 -> [DTC_raw44]
  DTCID45/1 -> DTCID+Status45/1
  [VOUTP_MCUF1NoComDTC_raw32] -> DTCID+Status45/2
  DTCID+Status45/1 -> [DTC_raw45]
  DTCID46/1 -> DTCID+Status46/1
  [VOUTP_Shifter1NoComDTC_raw32] -> DTCID+Status46/2
  DTCID+Status46/1 -> [DTC_raw46]
  DTCID47/1 -> DTCID+Status47/1
  [VOUTP_ESC1NoComDTC_raw32] -> DTCID+Status47/2
  DTCID+Status47/1 -> [DTC_raw47]
  DTCID48/1 -> DTCID+Status48/1
  [VOUTP_ESC5NoComDTC_raw32] -> DTCID+Status48/2
  DTCID+Status48/1 -> [DTC_raw48]
  DTCID49/1 -> DTCID+Status49/1
  [VOUTP_MCUR1RCErrDTC_raw32] -> DTCID+Status49/2
  DTCID+Status49/1 -> [DTC_raw49]
  DTCID50/1 -> DTCID+Status50/1
  [VOUTP_MCUF1RCErrDTC_raw32] -> DTCID+Status50/2
  DTCID+Status50/1 -> [DTC_raw50]
  DTCID51/1 -> DTCID+Status51/1
  [VOUTP_Shifter1RCErrDTC_raw32] -> DTCID+Status51/2
  DTCID+Status51/1 -> [DTC_raw51]
  DTCID52/1 -> DTCID+Status52/1
  [VOUTP_ESC1RCErrDTC_raw32] -> DTCID+Status52/2
  DTCID+Status52/1 -> [DTC_raw52]
  DTCID53/1 -> DTCID+Status53/1
  [VOUTP_ESC5RCErrDTC_raw32] -> DTCID+Status53/2
  DTCID+Status53/1 -> [DTC_raw53]
  DTCID54/1 -> DTCID+Status54/1
  [VOUTP_MCUR1CSErrDTC_raw32] -> DTCID+Status54/2
  DTCID+Status54/1 -> [DTC_raw54]
  DTCID55/1 -> DTCID+Status55/1
  [VOUTP_MCUF1CSErrDTC_raw32] -> DTCID+Status55/2
  DTCID+Status55/1 -> [DTC_raw55]
  DTCID56/1 -> DTCID+Status56/1
  [VOUTP_Shifter1CSErrDTC_raw32] -> DTCID+Status56/2
  DTCID+Status56/1 -> [DTC_raw56]
  DTCID57/1 -> DTCID+Status57/1
  [VOUTP_ESC1CSErrDTC_raw32] -> DTCID+Status57/2
  DTCID+Status57/1 -> [DTC_raw57]
  DTCID58/1 -> DTCID+Status58/1
  [VOUTP_ESC5CSErrDTC_raw32] -> DTCID+Status58/2
  DTCID+Status58/1 -> [DTC_raw58]
  DTCID59/1 -> DTCID+Status59/1
  [VOUTP_APS1SigOoRDTC_raw32] -> DTCID+Status59/2
  DTCID+Status59/1 -> [DTC_raw59]
  DTCID60/1 -> DTCID+Status60/1
  [VOUTP_APS2SigOoRDTC_raw32] -> DTCID+Status60/2
  DTCID+Status60/1 -> [DTC_raw60]
  DTCID61/1 -> DTCID+Status61/1
  [VOUTP_APSCorrErrDTC_raw32] -> DTCID+Status61/2
  DTCID+Status61/1 -> [DTC_raw61]
  DTCID62/1 -> DTCID+Status62/1
  [VOUTP_5vAPS1PwrErrDTC_raw32] -> DTCID+Status62/2
  DTCID+Status62/1 -> [DTC_raw62]
  DTCID63/1 -> DTCID+Status63/1
  [VOUTP_5vAPS2PwrErrDTC_raw32] -> DTCID+Status63/2
  DTCID+Status63/1 -> [DTC_raw63]
  DTCID64/1 -> DTCID+Status64/1
  [VOUTP_FrMCUTqErrDTC_raw32] -> DTCID+Status64/2
  DTCID+Status64/1 -> [DTC_raw64]
  DTCID65/1 -> DTCID+Status65/1
  [VOUTP_RrMCUTqErrDTC_raw32] -> DTCID+Status65/2
  DTCID+Status65/1 -> [DTC_raw65]
  DTCID66/1 -> DTCID+Status66/1
  [VOUTP_EPBLockTODTC_raw32] -> DTCID+Status66/2
  DTCID+Status66/1 -> [DTC_raw66]
  DTCID67/1 -> DTCID+Status67/1
  [VOUTP_EPBUnlockTODTC_raw32] -> DTCID+Status67/2
  DTCID+Status67/1 -> [DTC_raw67]
  DTCID68/1 -> DTCID+Status68/1
  [VOUTP_FCLUSSDTC_raw32] -> DTCID+Status68/2
  DTCID+Status68/1 -> [DTC_raw68]
  DTCID69/1 -> DTCID+Status69/1
  [VOUTP_FMLUSSDTC_raw32] -> DTCID+Status69/2
  DTCID+Status69/1 -> [DTC_raw69]
  DTCID70/1 -> DTCID+Status70/1
  [VOUTP_FMRUSSDTC_raw32] -> DTCID+Status70/2
  DTCID+Status70/1 -> [DTC_raw70]
  DTCID71/1 -> DTCID+Status71/1
  [VOUTP_FCRUSSDTC_raw32] -> DTCID+Status71/2
  DTCID+Status71/1 -> [DTC_raw71]
  DTCID72/1 -> DTCID+Status72/1
  [VOUTP_RCLUSSDTC_raw32] -> DTCID+Status72/2
  DTCID+Status72/1 -> [DTC_raw72]
  DTCID73/1 -> DTCID+Status73/1
  [VOUTP_RMLUSSDTC_raw32] -> DTCID+Status73/2
  DTCID+Status73/1 -> [DTC_raw73]
  DTCID74/1 -> DTCID+Status74/1
  [VOUTP_RMRUSSDTC_raw32] -> DTCID+Status74/2
  DTCID+Status74/1 -> [DTC_raw74]
  DTCID75/1 -> DTCID+Status75/1
  [VOUTP_RCRUSSDTC_raw32] -> DTCID+Status75/2
  DTCID+Status75/1 -> [DTC_raw75]
  DTCID76/1 -> DTCID+Status76/1
  [VOUTP_FLLUSSDTC_raw32] -> DTCID+Status76/2
  DTCID+Status76/1 -> [DTC_raw76]
  DTCID77/1 -> DTCID+Status77/1
  [VOUTP_FLRUSSDTC_raw32] -> DTCID+Status77/2
  DTCID+Status77/1 -> [DTC_raw77]
  DTCID78/1 -> DTCID+Status78/1
  [VOUTP_RLLUSSDTC_raw32] -> DTCID+Status78/2
  DTCID+Status78/1 -> [DTC_raw78]
  DTCID79/1 -> DTCID+Status79/1
  [VOUTP_RLRUSSDTC_raw32] -> DTCID+Status79/2
  DTCID+Status79/1 -> [DTC_raw79]
  DTCID80/1 -> DTCID+Status80/1
  [VOUTP_LFPressIndiDTC_raw32] -> DTCID+Status80/2
  DTCID+Status80/1 -> [DTC_raw80]
  DTCID81/1 -> DTCID+Status81/1
  [VOUTP_RFPressIndiDTC_raw32] -> DTCID+Status81/2
  DTCID+Status81/1 -> [DTC_raw81]
  DTCID82/1 -> DTCID+Status82/1
  [VOUTP_LRPressIndiDTC_raw32] -> DTCID+Status82/2
  DTCID+Status82/1 -> [DTC_raw82]
  DTCID83/1 -> DTCID+Status83/1
  [VOUTP_RRPressIndiDTC_raw32] -> DTCID+Status83/2
  DTCID+Status83/1 -> [DTC_raw83]
  DTCID84/1 -> DTCID+Status84/1
  [VOUTP_LFWheelTmpHighDTC_raw32] -> DTCID+Status84/2
  DTCID+Status84/1 -> [DTC_raw84]
  DTCID85/1 -> DTCID+Status85/1
  [VOUTP_RFWheelTmpHighDTC_raw32] -> DTCID+Status85/2
  DTCID+Status85/1 -> [DTC_raw85]
  DTCID86/1 -> DTCID+Status86/1
  [VOUTP_LRWheelTmpHighDTC_raw32] -> DTCID+Status86/2
  DTCID+Status86/1 -> [DTC_raw86]
  DTCID87/1 -> DTCID+Status87/1
  [VOUTP_RRWheelTmpHighDTC_raw32] -> DTCID+Status87/2
  DTCID+Status87/1 -> [DTC_raw87]
  DTCID88/1 -> DTCID+Status88/1
  [VOUTP_LFBatwarnDTC_raw32] -> DTCID+Status88/2
  DTCID+Status88/1 -> [DTC_raw88]
  DTCID89/1 -> DTCID+Status89/1
  [VOUTP_RFBatwarnDTC_raw32] -> DTCID+Status89/2
  DTCID+Status89/1 -> [DTC_raw89]
  DTCID90/1 -> DTCID+Status90/1
  [VOUTP_LRBatwarnDTC_raw32] -> DTCID+Status90/2
  DTCID+Status90/1 -> [DTC_raw90]
  DTCID91/1 -> DTCID+Status91/1
  [VOUTP_RRBatwarnDTC_raw32] -> DTCID+Status91/2
  DTCID+Status91/1 -> [DTC_raw91]
  DTCID92/1 -> DTCID+Status92/1
  [VOUTP_LFSensorFailDTC_raw32] -> DTCID+Status92/2
  DTCID+Status92/1 -> [DTC_raw92]
  DTCID93/1 -> DTCID+Status93/1
  [VOUTP_RFSensorFailDTC_raw32] -> DTCID+Status93/2
  DTCID+Status93/1 -> [DTC_raw93]
  DTCID94/1 -> DTCID+Status94/1
  [VOUTP_LRSensorFailDTC_raw32] -> DTCID+Status94/2
  DTCID+Status94/1 -> [DTC_raw94]
  DTCID95/1 -> DTCID+Status95/1
  [VOUTP_RRSensorFailDTC_raw32] -> DTCID+Status95/2
  DTCID+Status95/1 -> [DTC_raw95]
  DTCID96/1 -> DTCID+Status96/1
  [VOUTP_DiagFRTSDTC_raw32] -> DTCID+Status96/2
  DTCID+Status96/1 -> [DTC_raw96]
  DTCID97/1 -> DTCID+Status97/1
  [VOUTP_DiagRRTSDTC_raw32] -> DTCID+Status97/2
  DTCID+Status97/1 -> [DTC_raw97]
  DTCID98/1 -> DTCID+Status98/1
  [VOUTP_DiagFLTSDTC_raw32] -> DTCID+Status98/2
  DTCID+Status98/1 -> [DTC_raw98]
  DTCID99/1 -> DTCID+Status99/1
  [VOUTP_DiagRLTSDTC_raw32] -> DTCID+Status99/2
  DTCID+Status99/1 -> [DTC_raw99]
  DTCID100/1 -> DTCID+Status100/1
  [VOUTP_DiagHCrashDTC_raw32] -> DTCID+Status100/2
  DTCID+Status100/1 -> [DTC_raw100]
  DTCID101/1 -> DTCID+Status101/1
  [VOUTP_HoodSWDTC_raw32] -> DTCID+Status101/2
  DTCID+Status101/1 -> [DTC_raw101]
  DTCID102/1 -> DTCID+Status102/1
  [VOUTP_TailgaSWDTC_raw32] -> DTCID+Status102/2
  DTCID+Status102/1 -> [DTC_raw102]
  DTCID103/1 -> DTCID+Status103/1
  [VOUTP_BMSSigErrDetDTC_raw32] -> DTCID+Status103/2
  DTCID+Status103/1 -> [DTC_raw103]
  DTCID104/1 -> DTCID+Status104/1
  [VOUTP_FCMACCSigErrDetDTC_raw32] -> DTCID+Status104/2
  DTCID+Status104/1 -> [DTC_raw104]
  DTCID105/1 -> DTCID+Status105/1
  [VOUTP_FrMCUSigErrDetDTC_raw32] -> DTCID+Status105/2
  DTCID+Status105/1 -> [DTC_raw105]
  DTCID106/1 -> DTCID+Status106/1
  [VOUTP_RrMCUSigErrDetDTC_raw32] -> DTCID+Status106/2
  DTCID+Status106/1 -> [DTC_raw106]
  DTCID107/1 -> DTCID+Status107/1
  [VOUTP_CCUSigErrDetDTC_raw32] -> DTCID+Status107/2
  DTCID+Status107/1 -> [DTC_raw107]
  DTCID108/1 -> DTCID+Status108/1
  [VOUTP_ACCAccelCmdErrDetDTC_raw32] -> DTCID+Status108/2
  DTCID+Status108/1 -> [DTC_raw108]
  DTCID109/1 -> DTCID+Status109/1
  [VOUTP_CAN1BusErrorDTC_raw32] -> DTCID+Status109/2
  DTCID+Status109/1 -> [DTC_raw109]
  DTCID110/1 -> DTCID+Status110/1
  [VOUTP_CAN2BusErrorDTC_raw32] -> DTCID+Status110/2
  DTCID+Status110/1 -> [DTC_raw110]
  DTCID111/1 -> DTCID+Status111/1
  [VOUTP_CAN3BusErrorDTC_raw32] -> DTCID+Status111/2
  DTCID+Status111/1 -> [DTC_raw111]
  DTCID112/1 -> DTCID+Status112/1
  [VOUTP_CAN4BusErrorDTC_raw32] -> DTCID+Status112/2
  DTCID+Status112/1 -> [DTC_raw112]
  DTCID113/1 -> DTCID+Status113/1
  [VOUTP_CAN5BusErrorDTC_raw32] -> DTCID+Status113/2
  DTCID+Status113/1 -> [DTC_raw113]
  DTCID114/1 -> DTCID+Status114/1
  [VOUTP_CAN6BusErrorDTC_raw32] -> DTCID+Status114/2
  DTCID+Status114/1 -> [DTC_raw114]
  Constant/1 -> Mux/1
  Constant1/1 -> Mux/2
  Constant2/1 -> Mux/3
  Constant3/1 -> Mux/4
  Constant4/1 -> Mux/5
  Constant5/1 -> Mux/6
  Constant6/1 -> Mux/7
  Constant7/1 -> Mux/8
  Constant8/1 -> Mux/9
  Constant9/1 -> Mux/10
  Constant10/1 -> Mux/11
  Constant11/1 -> Mux/12
  Constant12/1 -> Mux/13
  Constant13/1 -> Mux/14
  Constant14/1 -> Mux/15
  Constant15/1 -> Mux/16
  Constant16/1 -> Mux/17
  Constant17/1 -> Mux/18
  Constant18/1 -> Mux/19
  Constant19/1 -> Mux/20
  Constant20/1 -> Mux/21
  Constant21/1 -> Mux/22
  Constant22/1 -> Mux/23
  Constant23/1 -> Mux/24
  Constant24/1 -> Mux/25
  Constant25/1 -> Mux/26
  Constant26/1 -> Mux/27
  Constant27/1 -> Mux/28
  Constant28/1 -> Mux/29
  Constant29/1 -> Mux/30
  Constant30/1 -> Mux/31
  Constant31/1 -> Mux/32
  Constant32/1 -> Mux/33
  Constant33/1 -> Mux/34
  Constant34/1 -> Mux/35
  Constant35/1 -> Mux/36
  Constant36/1 -> Mux/37
  Constant37/1 -> Mux/38
  Constant38/1 -> Mux/39
  Constant39/1 -> Mux/40
  Constant40/1 -> Mux/41
  Constant41/1 -> Mux/42
  Constant42/1 -> Mux/43
  Constant43/1 -> Mux/44
  Constant44/1 -> Mux/45
  Constant45/1 -> Mux/46
  Constant46/1 -> Mux/47
  Constant47/1 -> Mux/48
  Constant48/1 -> Mux/49
  Constant49/1 -> Mux/50
  Constant50/1 -> Mux/51
  Constant51/1 -> Mux/52
  Constant52/1 -> Mux/53
  Constant53/1 -> Mux/54
  Constant54/1 -> Mux/55
  Constant55/1 -> Mux/56
  Constant56/1 -> Mux/57
  Constant57/1 -> Mux/58
  Constant58/1 -> Mux/59
  Constant59/1 -> Mux/60
  Constant60/1 -> Mux/61
  Constant61/1 -> Mux/62
  Constant62/1 -> Mux/63
  Constant63/1 -> Mux/64
  Constant64/1 -> Mux/65
  Constant65/1 -> Mux/66
  Constant66/1 -> Mux/67
  Constant67/1 -> Mux/68
  Constant68/1 -> Mux/69
  Constant69/1 -> Mux/70
  Constant70/1 -> Mux/71
  Constant71/1 -> Mux/72
  Constant72/1 -> Mux/73
  Constant73/1 -> Mux/74
  Constant74/1 -> Mux/75
  Constant75/1 -> Mux/76
  Constant76/1 -> Mux/77
  Constant77/1 -> Mux/78
  Constant78/1 -> Mux/79
  Constant79/1 -> Mux/80
  Constant80/1 -> Mux/81
  Constant81/1 -> Mux/82
  Constant82/1 -> Mux/83
  Constant83/1 -> Mux/84
  Constant84/1 -> Mux/85
  Constant85/1 -> Mux/86
  Constant86/1 -> Mux/87
  Constant87/1 -> Mux/88
  Constant88/1 -> Mux/89
  Constant89/1 -> Mux/90
  Constant90/1 -> Mux/91
  Constant91/1 -> Mux/92
  Constant92/1 -> Mux/93
  Constant93/1 -> Mux/94
  Constant94/1 -> Mux/95
  Constant95/1 -> Mux/96
  Constant96/1 -> Mux/97
  Constant97/1 -> Mux/98
  Constant98/1 -> Mux/99
  Constant99/1 -> Mux/100
  Constant100/1 -> Mux/101
  Constant101/1 -> Mux/102
  Constant102/1 -> Mux/103
  Constant103/1 -> Mux/104
  Constant104/1 -> Mux/105
  Constant105/1 -> Mux/106
  Constant106/1 -> Mux/107
  Constant107/1 -> Mux/108
  Constant108/1 -> Mux/109
  Constant109/1 -> Mux/110
  Constant110/1 -> Mux/111
  Constant111/1 -> Mux/112
  Constant112/1 -> Mux/113
  Constant113/1 -> Mux/114
  Constant114/1 -> Mux/115
  Mux/1 -> Mux1/1
  Constant115/1 -> Mux1/2
  Mux1/1 -> Constant116/1, DTC_Constant_Array/1
  Constant116/1 -> [DTC_Constant_Array]
  [DTC_raw0] -> Mux2/1
  [DTC_raw1] -> Mux2/2
  [DTC_raw2] -> Mux2/3
  [DTC_raw3] -> Mux2/4
  [DTC_raw4] -> Mux2/5
  [DTC_raw5] -> Mux2/6
  [DTC_raw6] -> Mux2/7
  [DTC_raw7] -> Mux2/8
  [DTC_raw8] -> Mux2/9
  [DTC_raw9] -> Mux2/10
  [DTC_raw10] -> Mux2/11
  [DTC_raw11] -> Mux2/12
  [DTC_raw12] -> Mux2/13
  [DTC_raw13] -> Mux2/14
  [DTC_raw14] -> Mux2/15
  [DTC_raw15] -> Mux2/16
  [DTC_raw16] -> Mux2/17
  [DTC_raw17] -> Mux2/18
  [DTC_raw18] -> Mux2/19
  [DTC_raw19] -> Mux2/20
  [DTC_raw20] -> Mux2/21
  [DTC_raw21] -> Mux2/22
  [DTC_raw22] -> Mux2/23
  [DTC_raw23] -> Mux2/24
  [DTC_raw24] -> Mux2/25
  [DTC_raw25] -> Mux2/26
  [DTC_raw26] -> Mux2/27
  [DTC_raw27] -> Mux2/28
  [DTC_raw28] -> Mux2/29
  [DTC_raw29] -> Mux2/30
  [DTC_raw30] -> Mux2/31
  [DTC_raw31] -> Mux2/32
  [DTC_raw32] -> Mux2/33
  [DTC_raw33] -> Mux2/34
  [DTC_raw34] -> Mux2/35
  [DTC_raw35] -> Mux2/36
  [DTC_raw36] -> Mux2/37
  [DTC_raw37] -> Mux2/38
  [DTC_raw38] -> Mux2/39
  [DTC_raw39] -> Mux2/40
  [DTC_raw40] -> Mux2/41
  [DTC_raw41] -> Mux2/42
  [DTC_raw42] -> Mux2/43
  [DTC_raw43] -> Mux2/44
  [DTC_raw44] -> Mux2/45
  [DTC_raw45] -> Mux2/46
  [DTC_raw46] -> Mux2/47
  [DTC_raw47] -> Mux2/48
  [DTC_raw48] -> Mux2/49
  [DTC_raw49] -> Mux2/50
  [DTC_raw50] -> Mux2/51
  [DTC_raw51] -> Mux2/52
  [DTC_raw52] -> Mux2/53
  [DTC_raw53] -> Mux2/54
  [DTC_raw54] -> Mux2/55
  [DTC_raw55] -> Mux2/56
  [DTC_raw56] -> Mux2/57
  [DTC_raw57] -> Mux2/58
  [DTC_raw58] -> Mux2/59
  [DTC_raw59] -> Mux2/60
  [DTC_raw60] -> Mux2/61
  [DTC_raw61] -> Mux2/62
  [DTC_raw62] -> Mux2/63
  [DTC_raw63] -> Mux2/64
  [DTC_raw64] -> Mux2/65
  [DTC_raw65] -> Mux2/66
  [DTC_raw66] -> Mux2/67
  [DTC_raw67] -> Mux2/68
  [DTC_raw68] -> Mux2/69
  [DTC_raw69] -> Mux2/70
  [DTC_raw70] -> Mux2/71
  [DTC_raw71] -> Mux2/72
  [DTC_raw72] -> Mux2/73
  [DTC_raw73] -> Mux2/74
  [DTC_raw74] -> Mux2/75
  [DTC_raw75] -> Mux2/76
  [DTC_raw76] -> Mux2/77
  [DTC_raw77] -> Mux2/78
  [DTC_raw78] -> Mux2/79
  [DTC_raw79] -> Mux2/80
  [DTC_raw80] -> Mux2/81
  [DTC_raw81] -> Mux2/82
  [DTC_raw82] -> Mux2/83
  [DTC_raw83] -> Mux2/84
  [DTC_raw84] -> Mux2/85
  [DTC_raw85] -> Mux2/86
  [DTC_raw86] -> Mux2/87
  [DTC_raw87] -> Mux2/88
  [DTC_raw88] -> Mux2/89
  [DTC_raw89] -> Mux2/90
  [DTC_raw90] -> Mux2/91
  [DTC_raw91] -> Mux2/92
  [DTC_raw92] -> Mux2/93
  [DTC_raw93] -> Mux2/94
  [DTC_raw94] -> Mux2/95
  [DTC_raw95] -> Mux2/96
  [DTC_raw96] -> Mux2/97
  [DTC_raw97] -> Mux2/98
  [DTC_raw98] -> Mux2/99
  [DTC_raw99] -> Mux2/100
  [DTC_raw100] -> Mux2/101
  [DTC_raw101] -> Mux2/102
  [DTC_raw102] -> Mux2/103
  [DTC_raw103] -> Mux2/104
  [DTC_raw104] -> Mux2/105
  [DTC_raw105] -> Mux2/106
  [DTC_raw106] -> Mux2/107
  [DTC_raw107] -> Mux2/108
  [DTC_raw108] -> Mux2/109
  [DTC_raw109] -> Mux2/110
  [DTC_raw110] -> Mux2/111
  [DTC_raw111] -> Mux2/112
  [DTC_raw112] -> Mux2/113
  [DTC_raw113] -> Mux2/114
  [DTC_raw114] -> Mux2/115
  Mux2/1 -> Mux3/1
  Constant117/1 -> Mux3/2
  Mux3/1 -> Constant118/1, DTC_Array/1
  Constant118/1 -> [DTC_Array]  "VDTC_DTCArray_raw32"
  [DTC_Array] -> BitwiseAND/1
  BitwiseAND/1 -> detect_change/1
  detect_change/1 -> Selector8/1, Selector9/1, Selector7/1, Selector6/1, Selector5/1, Selector4/1, Selector3/1, Selector2/1, Selector1/1, Selector/1
  Selector/1 -> DTCHeader/1
  DTCHeader/1 -> Mux4/1
  Selector1/1 -> DTCHeader1/1
  DTCHeader1/1 -> Mux4/2
  Selector2/1 -> DTCHeader2/1
  DTCHeader2/1 -> Mux4/3
  Selector3/1 -> DTCHeader3/1
  DTCHeader3/1 -> Mux4/4
  Selector4/1 -> DTCHeader4/1
  DTCHeader4/1 -> Mux4/5
  Selector5/1 -> DTCHeader5/1
  DTCHeader5/1 -> Mux4/6
  Selector6/1 -> DTCHeader6/1
  DTCHeader6/1 -> Mux4/7
  Selector7/1 -> DTCHeader7/1
  DTCHeader7/1 -> Mux4/8
  Selector8/1 -> DTCHeader8/1
  DTCHeader8/1 -> Mux4/9
  Selector9/1 -> DTCHeader9/1
  DTCHeader9/1 -> Mux4/10
  Mux4/1 -> UnitConverter/1, OR/1
  UnitConverter/1 -> Header_Array/1  "VDTC_HeaderArray_raw32"
  OR/1 -> Trigger/1  "VHAL_TriggerDTC_flg"
